simulink model "Battery_charge_discharge_FSBB_DCDC"  (R2022b)
settings: Solver=ode23tb  StartTime=0.0  StopTime=1.5  RelTol=1e-3  EnableMultiTasking=on
values from neighbouring files (symbols this model uses):
  time_step = 1 / wave_freq    (= 1.11111111111e-05)    [Battery_charge_discharge_FSBB_param_init.m]
undefined symbols (not defined in the file or in its folder): Ion, Lithium
libraries: spsTriangleGeneratorLib x13, spsSeriesRLCBranchLib x9, slpidlib x9, spsVoltageMeasurementLib x5, spsCurrentMeasurementLib x4, spsIGBTDiodeLib x4, spsBatteryLib x2, spsIdealSwitchLib x2, spsDCVoltageSourceLib x2, spsControlledVoltageSourceLib x1, spspowerguiLib x1
(part 2 of 2)

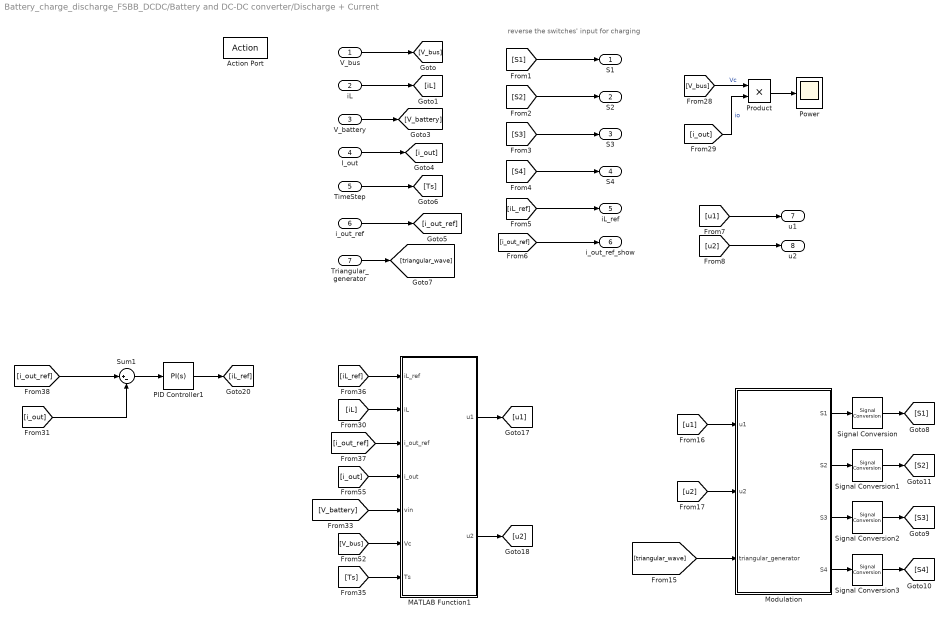
== system Battery_charge_discharge_FSBB_DCDC/Battery and DC-DC converter/Discharge + Current ==
  note: reverse the switches' input for charging
  V_bus : Inport
  iL : Inport  Port=2
  V_battery : Inport  Port=3
  I_out : Inport  Port=4
  TimeStep : Inport  Port=5
  i_out_ref : Inport  Port=6
  Triangular_generator : Inport  Port=7
  Action Port : ActionPort  ActionPortLabel=elseif( u1==1 & u2==1)
  MATLAB Function1 : MATLAB Function  TreatAsAtomicUnit=on
  Modulation : Subsystem
  PID Controller1 : slpidlib/PID Controller  Controller=PI  Form=Parallel  TimeDomain=Continuous-time  UseExternalTs=off  SampleTime=-1  IntegratorMethod=Forward Euler  FilterMethod=Forward Euler  ControllerParametersSource=internal  P=15  I=1000  UseKiTs=on  D=0  N=100  UseFilter=on  TunerSelectOption=Transfer Function Based (PID Tuner App)  InitialConditionSource=internal  InitialConditionForIntegrator=0  InitialConditionForFilter=0  DifferentiatorICPrevScaledInput=0  ExternalReset=none  TrackingMode=off  Kt=1  LimitOutput=on  SatLimitsSource=internal  UpperSaturationLimit=50  LowerSaturationLimit=-10  LinearizeAsGain=on  AntiWindupMode=none  Kb=1  LimitIntegrator=off  UpperIntegratorSaturationLimit=inf  LowerIntegratorSaturationLimit=-inf  POutMin=[]  POutMax=[]  IOutMin=[]  IOutMax=[]  DOutMin=[]  DOutMax=[]  NOutMin=[]  NOutMax=[]  SumOutMin=[]  SumOutMax=[]  SaturationOutMin=[]  SaturationOutMax=[]  PParamMin=[]  PParamMax=[]  IParamMin=[]  IParamMax=[]  DParamMin=[]  DParamMax=[]  NParamMin=[]  NParamMax=[]  KbParamMin=[]  KbParamMax=[]  KtParamMin=[]  KtParamMax=[]  KbOutMin=[]  KbOutMax=[]  KtOutMin=[]  KtOutMax=[]  IntegratorOutMin=[]  IntegratorOutMax=[]  FilterOutMin=[]  FilterOutMax=[]  SumI1OutMin=[]  SumI1OutMax=[]  SumI2OutMin=[]  SumI2OutMax=[]  SumI3OutMin=[]  SumI3OutMax=[]  SumI4OutMin=[]  SumI4OutMax=[]  SumDOutMin=[]  SumDOutMax=[]  DifferentiatorOutMin=[]  DifferentiatorOutMax=[]  FilterDiffOutCoefMin=[]  FilterDiffOutCoefMax=[]  ReciprocalOutMin=[]  ReciprocalOutMax=[]  SumDenOutMin=[]  SumDenOutMax=[]  SumNumOutMin=[]  SumNumOutMax=[]  DivideOutMin=[]  DivideOutMax=[]  UdiffTsProdOutMin=[]  UdiffTsProdOutMax=[]  NTsProdOutMin=[]  NTsProdOutMax=[]  UintegralTsProdOutMin=[]  UintegralTsProdOutMax=[]  UngainTsProdOutMin=[]  UngainTsProdOutMax=[]  ClampingZeroOutDataTypeStr=Inherit: Inherit via back propagation  ClampingZeroOutMin=[]  ClampingZeroOutMax=[]  FilterDenConstantOutDataTypeStr=Inherit: Inherit via back propagation  FilterDenConstantOutMin=[]  FilterDenConstantOutMax=[]  PCopyOutDataTypeStr=Inherit: Inherit via back propagation  PCopyOutMin=[]  PCopyOutMax=[]  NCopyOutDataTypeStr=Inherit: Inherit via back propagation  NCopyOutMin=[]  NCopyOutMax=[]  IntegratorContinuousStateAttributes=''  IntegratorStateMustResolveToSignalObject=off  IntegratorRTWStateStorageClass=Auto  FilterContinuousStateAttributes=''  FilterStateMustResolveToSignalObject=off  FilterRTWStateStorageClass=Auto  ParallelPVariant=InternalParameters  IdealPVariant=Disabled  IVariant=InternalParameters  DVariant=Disabled  IntegratorVariant=Continuous  SatVariant=Enabled  AWVariant=Passthrough  PCopyVariant=Disabled  TRVariant=Disabled  FdbkBlocksVariant=Forward  IdealPFdbkVariant=Disabled  SatFdbkVariant=Disabled  DerivativeFilterVariant=Disabled  NVariant=Disabled  NCopyVariant=Disabled_SignalSpec  FilterICVariant=Disabled  IntegratorICVariant=InternalICs  ExternalResetVariant=Disabled  TRSumVariant=Passthrough  SumFdbkVariant=Disabled  SumVariant=Sum_PI  TsampFilterVariant=InternalTs  TsampNgainVariant=Passthrough  TsampIntegralVariant=Passthrough  ExternalSaturationOutDataTypeStr=Inherit: Same as second input
  Power : Scope
  Product : Product
  Signal Conversion{,1..3} (4 alike) : SignalConversion  OverrideOpt=off
  Sum1 : Sum  Inputs=|+-
  S1 : Outport
  S2 : Outport  Port=2
  S3 : Outport  Port=3
  S4 : Outport  Port=4
  iL_ref : Outport  Port=5
  i_out_ref_show : Outport  Port=6
  u1 : Outport  Port=7
  u2 : Outport  Port=8
  wires:
  Modulation/2(S2) -> Signal Conversion1/1
  Modulation/1(S1) -> Signal Conversion/1
  Modulation/3(S3) -> Signal Conversion2/1
  [u1] -> Modulation/1(u1)
  [i_out] -> Product/2  "io"
  [u2] -> Modulation/2(u2)
  [V_bus] -> Product/1  "Vc"
  Product/1 -> Power/1
  Modulation/4(S4) -> Signal Conversion3/1
  V_bus/1 -> [V_bus]
  iL/1 -> [iL]
  V_battery/1 -> [V_battery]
  I_out/1 -> [i_out]
  TimeStep/1 -> [Ts]
  i_out_ref/1 -> [i_out_ref]
  [iL_ref] -> iL_ref/1
  [i_out_ref] -> i_out_ref_show/1
  [u2] -> u2/1
  [u1] -> u1/1
  [triangular_wave] -> Modulation/3(triangular_generator)
  Triangular_generator/1 -> [triangular_wave]
  Signal Conversion/1 -> [S1]
  Signal Conversion1/1 -> [S2]
  Signal Conversion2/1 -> [S3]
  Signal Conversion3/1 -> [S4]
  [iL] -> MATLAB Function1/2(iL)
  Sum1/1 -> PID Controller1/1
  [i_out] -> Sum1/2
  [i_out] -> MATLAB Function1/4(i_out)
  [V_bus] -> MATLAB Function1/6(Vc)
  [Ts] -> MATLAB Function1/7(Ts)
  PID Controller1/1 -> [iL_ref]
  MATLAB Function1/2(u2) -> [u2]
  MATLAB Function1/1(u1) -> [u1]
  [i_out_ref] -> Sum1/1
  [i_out_ref] -> MATLAB Function1/3(i_out_ref)
  [iL_ref] -> MATLAB Function1/1(iL_ref)
  [V_battery] -> MATLAB Function1/5(vin)
  [S1] -> S1/1
  [S3] -> S3/1
  [S4] -> S4/1
  [S2] -> S2/1

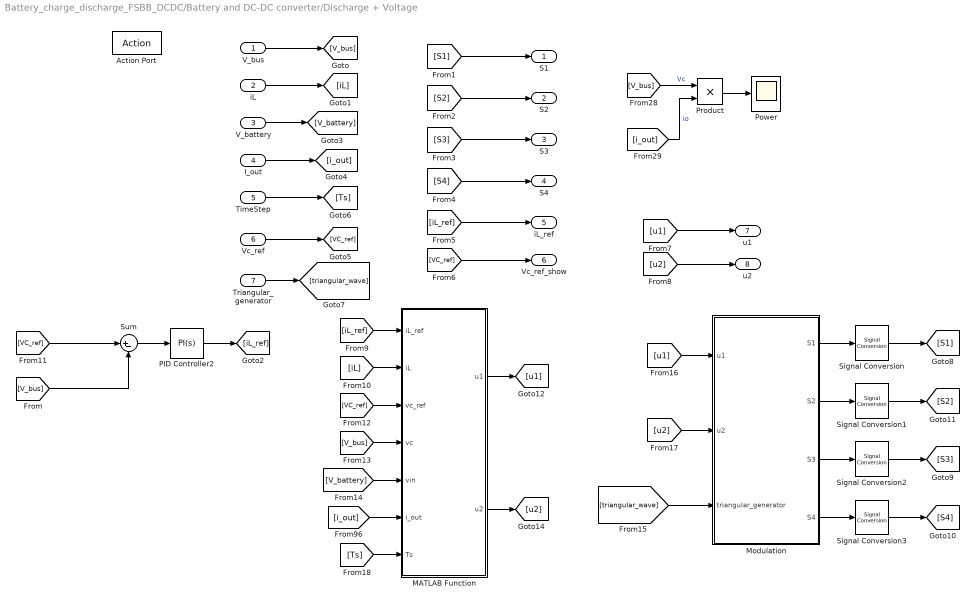
== system Battery_charge_discharge_FSBB_DCDC/Battery and DC-DC converter/Discharge + Voltage ==
  V_bus : Inport
  iL : Inport  Port=2
  V_battery : Inport  Port=3
  I_out : Inport  Port=4
  TimeStep : Inport  Port=5
  Vc_ref : Inport  Port=6
  Triangular_generator : Inport  Port=7
  Action Port : ActionPort  ActionPortLabel=if(u1 == 1 & u2 ==0)
  MATLAB Function : MATLAB Function  TreatAsAtomicUnit=on
  Modulation : Subsystem
  PID Controller2 : slpidlib/PID Controller  Controller=PI  Form=Parallel  TimeDomain=Continuous-time  UseExternalTs=off  SampleTime=-1  IntegratorMethod=Forward Euler  FilterMethod=Forward Euler  ControllerParametersSource=internal  P=15  I=1000  UseKiTs=on  D=0  N=100  UseFilter=on  TunerSelectOption=Transfer Function Based (PID Tuner App)  InitialConditionSource=internal  InitialConditionForIntegrator=0  InitialConditionForFilter=0  DifferentiatorICPrevScaledInput=0  ExternalReset=none  TrackingMode=off  Kt=1  LimitOutput=on  SatLimitsSource=internal  UpperSaturationLimit=50  LowerSaturationLimit=-10  LinearizeAsGain=on  AntiWindupMode=none  Kb=1  LimitIntegrator=off  UpperIntegratorSaturationLimit=inf  LowerIntegratorSaturationLimit=-inf  POutMin=[]  POutMax=[]  IOutMin=[]  IOutMax=[]  DOutMin=[]  DOutMax=[]  NOutMin=[]  NOutMax=[]  SumOutMin=[]  SumOutMax=[]  SaturationOutMin=[]  SaturationOutMax=[]  PParamMin=[]  PParamMax=[]  IParamMin=[]  IParamMax=[]  DParamMin=[]  DParamMax=[]  NParamMin=[]  NParamMax=[]  KbParamMin=[]  KbParamMax=[]  KtParamMin=[]  KtParamMax=[]  KbOutMin=[]  KbOutMax=[]  KtOutMin=[]  KtOutMax=[]  IntegratorOutMin=[]  IntegratorOutMax=[]  FilterOutMin=[]  FilterOutMax=[]  SumI1OutMin=[]  SumI1OutMax=[]  SumI2OutMin=[]  SumI2OutMax=[]  SumI3OutMin=[]  SumI3OutMax=[]  SumI4OutMin=[]  SumI4OutMax=[]  SumDOutMin=[]  SumDOutMax=[]  DifferentiatorOutMin=[]  DifferentiatorOutMax=[]  FilterDiffOutCoefMin=[]  FilterDiffOutCoefMax=[]  ReciprocalOutMin=[]  ReciprocalOutMax=[]  SumDenOutMin=[]  SumDenOutMax=[]  SumNumOutMin=[]  SumNumOutMax=[]  DivideOutMin=[]  DivideOutMax=[]  UdiffTsProdOutMin=[]  UdiffTsProdOutMax=[]  NTsProdOutMin=[]  NTsProdOutMax=[]  UintegralTsProdOutMin=[]  UintegralTsProdOutMax=[]  UngainTsProdOutMin=[]  UngainTsProdOutMax=[]  ClampingZeroOutDataTypeStr=Inherit: Inherit via back propagation  ClampingZeroOutMin=[]  ClampingZeroOutMax=[]  FilterDenConstantOutDataTypeStr=Inherit: Inherit via back propagation  FilterDenConstantOutMin=[]  FilterDenConstantOutMax=[]  PCopyOutDataTypeStr=Inherit: Inherit via back propagation  PCopyOutMin=[]  PCopyOutMax=[]  NCopyOutDataTypeStr=Inherit: Inherit via back propagation  NCopyOutMin=[]  NCopyOutMax=[]  IntegratorContinuousStateAttributes=''  IntegratorStateMustResolveToSignalObject=off  IntegratorRTWStateStorageClass=Auto  FilterContinuousStateAttributes=''  FilterStateMustResolveToSignalObject=off  FilterRTWStateStorageClass=Auto  ParallelPVariant=InternalParameters  IdealPVariant=Disabled  IVariant=InternalParameters  DVariant=Disabled  IntegratorVariant=Continuous  SatVariant=Enabled  AWVariant=Passthrough  PCopyVariant=Disabled  TRVariant=Disabled  FdbkBlocksVariant=Forward  IdealPFdbkVariant=Disabled  SatFdbkVariant=Disabled  DerivativeFilterVariant=Disabled  NVariant=Disabled  NCopyVariant=Disabled_SignalSpec  FilterICVariant=Disabled  IntegratorICVariant=InternalICs  ExternalResetVariant=Disabled  TRSumVariant=Passthrough  SumFdbkVariant=Disabled  SumVariant=Sum_PI  TsampFilterVariant=InternalTs  TsampNgainVariant=Passthrough  TsampIntegralVariant=Passthrough  ExternalSaturationOutDataTypeStr=Inherit: Same as second input
  Power : Scope
  Product : Product
  Signal Conversion{,1..3} (4 alike) : SignalConversion  OverrideOpt=off
  Sum : Sum  Inputs=|+-
  S1 : Outport
  S2 : Outport  Port=2
  S3 : Outport  Port=3
  S4 : Outport  Port=4
  iL_ref : Outport  Port=5
  Vc_ref_show : Outport  Port=6
  u1 : Outport  Port=7
  u2 : Outport  Port=8
  wires:
  PID Controller2/1 -> [iL_ref]
  Modulation/2(S2) -> Signal Conversion1/1
  [Ts] -> MATLAB Function/7(Ts)
  Modulation/1(S1) -> Signal Conversion/1
  Sum/1 -> PID Controller2/1
  Modulation/3(S3) -> Signal Conversion2/1
  MATLAB Function/2(u2) -> [u2]
  [V_bus] -> MATLAB Function/4(vc)
  [u1] -> Modulation/1(u1)
  [VC_ref] -> Sum/1
  [VC_ref] -> MATLAB Function/3(vc_ref)
  MATLAB Function/1(u1) -> [u1]
  [i_out] -> Product/2  "io"
  [u2] -> Modulation/2(u2)
  [i_out] -> MATLAB Function/6(i_out)
  [iL] -> MATLAB Function/2(iL)
  [V_battery] -> MATLAB Function/5(vin)
  [V_bus] -> Product/1  "Vc"
  [iL_ref] -> MATLAB Function/1(iL_ref)
  Product/1 -> Power/1
  Modulation/4(S4) -> Signal Conversion3/1
  V_bus/1 -> [V_bus]
  [V_bus] -> Sum/2
  iL/1 -> [iL]
  V_battery/1 -> [V_battery]
  I_out/1 -> [i_out]
  TimeStep/1 -> [Ts]
  [S1] -> S1/1
  [S2] -> S2/1
  [S4] -> S4/1
  [S3] -> S3/1
  Vc_ref/1 -> [VC_ref]
  [iL_ref] -> iL_ref/1
  [VC_ref] -> Vc_ref_show/1
  [u2] -> u2/1
  [u1] -> u1/1
  [triangular_wave] -> Modulation/3(triangular_generator)
  Triangular_generator/1 -> [triangular_wave]
  Signal Conversion/1 -> [S1]
  Signal Conversion1/1 -> [S2]
  Signal Conversion2/1 -> [S3]
  Signal Conversion3/1 -> [S4]

== system Battery_charge_discharge_FSBB_DCDC/Battery and DC-DC converter/If Action Subsystem ==
  Action Port : ActionPort  ActionPortLabel=else
  Constant : Constant
  Stop Simulation : Stop
  wires:
  Constant/1 -> Stop Simulation/1

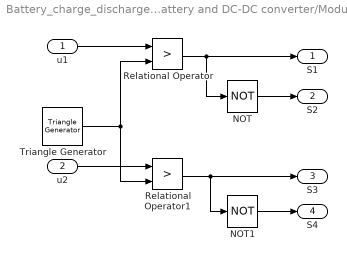
== system Battery_charge_discharge_FSBB_DCDC/Battery and DC-DC converter/Modulation ==
  u1 : Inport
  u2 : Inport  Port=2
  NOT : Logic  Operator=NOT  AllPortsSameDT=off  OutDataTypeStr=boolean
  NOT1 : Logic  Operator=NOT  AllPortsSameDT=off  OutDataTypeStr=boolean
  Relational Operator : RelationalOperator  Operator=>  OutDataTypeStr=boolean  RndMeth=Simplest  InputSameDT=off
  Relational Operator1 : RelationalOperator  Operator=>  OutDataTypeStr=boolean  RndMeth=Simplest  InputSameDT=off
  Triangle Generator : spsTriangleGeneratorLib/Triangle Generator  Freq=wave_freq  Phase=0  Ts=0
  S1 : Outport
  S2 : Outport  Port=2
  S3 : Outport  Port=3
  S4 : Outport  Port=4
  wires:
  u1/1 -> Relational Operator/1
  Triangle Generator/1 -> Relational Operator1/2, Relational Operator/2
  u2/1 -> Relational Operator1/1
  Relational Operator/1 -> NOT/1, S1/1
  NOT/1 -> S2/1
  Relational Operator1/1 -> NOT1/1, S3/1
  NOT1/1 -> S4/1

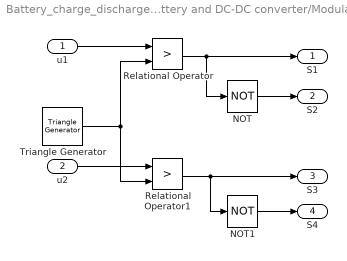
== system Battery_charge_discharge_FSBB_DCDC/Battery and DC-DC converter/Modulation1 ==
  u1 : Inport
  u2 : Inport  Port=2
  NOT : Logic  Operator=NOT  AllPortsSameDT=off  OutDataTypeStr=boolean
  NOT1 : Logic  Operator=NOT  AllPortsSameDT=off  OutDataTypeStr=boolean
  Relational Operator : RelationalOperator  Operator=>  OutDataTypeStr=boolean  RndMeth=Simplest  InputSameDT=off
  Relational Operator1 : RelationalOperator  Operator=>  OutDataTypeStr=boolean  RndMeth=Simplest  InputSameDT=off
  Triangle Generator : spsTriangleGeneratorLib/Triangle Generator  Freq=wave_freq  Phase=0  Ts=0
  S1 : Outport
  S2 : Outport  Port=2
  S3 : Outport  Port=3
  S4 : Outport  Port=4
  wires:
  u1/1 -> Relational Operator/1
  Triangle Generator/1 -> Relational Operator1/2, Relational Operator/2
  u2/1 -> Relational Operator1/1
  Relational Operator/1 -> NOT/1, S1/1
  NOT/1 -> S2/1
  Relational Operator1/1 -> NOT1/1, S3/1
  NOT1/1 -> S4/1

== system Battery_charge_discharge_FSBB_DCDC/Battery and DC-DC converter/Modulation2 ==
  u1 : Inport
  u2 : Inport  Port=2
  NOT : Logic  Operator=NOT  AllPortsSameDT=off  OutDataTypeStr=boolean
  NOT1 : Logic  Operator=NOT  AllPortsSameDT=off  OutDataTypeStr=boolean
  Relational Operator : RelationalOperator  Operator=>  OutDataTypeStr=boolean  RndMeth=Simplest  InputSameDT=off
  Relational Operator1 : RelationalOperator  Operator=>  OutDataTypeStr=boolean  RndMeth=Simplest  InputSameDT=off
  Triangle Generator : spsTriangleGeneratorLib/Triangle Generator  Freq=wave_freq  Phase=0  Ts=0
  S1 : Outport
  S2 : Outport  Port=2
  S3 : Outport  Port=3
  S4 : Outport  Port=4
  wires:
  u1/1 -> Relational Operator/1
  Triangle Generator/1 -> Relational Operator1/2, Relational Operator/2
  u2/1 -> Relational Operator1/1
  Relational Operator/1 -> NOT/1, S1/1
  NOT/1 -> S2/1
  Relational Operator1/1 -> NOT1/1, S3/1
  NOT1/1 -> S4/1

== system Battery_charge_discharge_FSBB_DCDC/Battery and DC-DC converter/Modulation3 ==
  u1 : Inport
  u2 : Inport  Port=2
  NOT : Logic  Operator=NOT  AllPortsSameDT=off  OutDataTypeStr=boolean
  NOT1 : Logic  Operator=NOT  AllPortsSameDT=off  OutDataTypeStr=boolean
  Relational Operator : RelationalOperator  Operator=>  OutDataTypeStr=boolean  RndMeth=Simplest  InputSameDT=off
  Relational Operator1 : RelationalOperator  Operator=>  OutDataTypeStr=boolean  RndMeth=Simplest  InputSameDT=off
  Triangle Generator : spsTriangleGeneratorLib/Triangle Generator  Freq=wave_freq  Phase=0  Ts=0
  S1 : Outport
  S2 : Outport  Port=2
  S3 : Outport  Port=3
  S4 : Outport  Port=4
  wires:
  u1/1 -> Relational Operator/1
  Triangle Generator/1 -> Relational Operator1/2, Relational Operator/2
  u2/1 -> Relational Operator1/1
  Relational Operator/1 -> NOT/1, S1/1
  NOT/1 -> S2/1
  Relational Operator1/1 -> NOT1/1, S3/1
  NOT1/1 -> S4/1

== system Battery_charge_discharge_FSBB_DCDC/Battery and DC-DC converter/Modulation5 ==
  u1 : Inport
  u2 : Inport  Port=2
  NOT : Logic  Operator=NOT  AllPortsSameDT=off  OutDataTypeStr=boolean
  NOT1 : Logic  Operator=NOT  AllPortsSameDT=off  OutDataTypeStr=boolean
  Relational Operator : RelationalOperator  Operator=>  OutDataTypeStr=boolean  RndMeth=Simplest  InputSameDT=off
  Relational Operator1 : RelationalOperator  Operator=>  OutDataTypeStr=boolean  RndMeth=Simplest  InputSameDT=off
  Triangle Generator : spsTriangleGeneratorLib/Triangle Generator  Freq=wave_freq  Phase=0  Ts=0
  S1 : Outport
  S2 : Outport  Port=2
  S3 : Outport  Port=3
  S4 : Outport  Port=4
  wires:
  u1/1 -> Relational Operator/1
  Triangle Generator/1 -> Relational Operator1/2, Relational Operator/2
  u2/1 -> Relational Operator1/1
  Relational Operator/1 -> NOT/1, S1/1
  NOT/1 -> S2/1
  Relational Operator1/1 -> NOT1/1, S3/1
  NOT1/1 -> S4/1

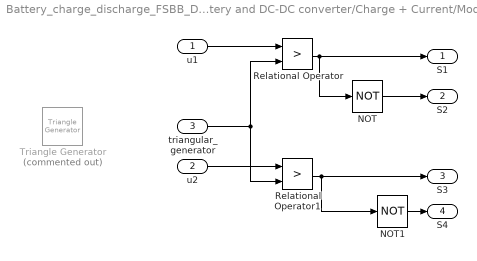
== system Battery_charge_discharge_FSBB_DCDC/Battery and DC-DC converter/Charge + Current/Modulation ==
  u1 : Inport
  u2 : Inport  Port=2
  triangular_generator : Inport  Port=3
  NOT : Logic  Operator=NOT  AllPortsSameDT=off  OutDataTypeStr=boolean
  NOT1 : Logic  Operator=NOT  AllPortsSameDT=off  OutDataTypeStr=boolean
  Relational Operator : RelationalOperator  Operator=>  OutDataTypeStr=boolean  RndMeth=Simplest  InputSameDT=off
  Relational Operator1 : RelationalOperator  Operator=>  OutDataTypeStr=boolean  RndMeth=Simplest  InputSameDT=off
  Triangle Generator : spsTriangleGeneratorLib/Triangle Generator  Commented=on  Freq=wave_freq  Phase=0  Ts=0
  S1 : Outport
  S2 : Outport  Port=2
  S3 : Outport  Port=3
  S4 : Outport  Port=4
  wires:
  u1/1 -> Relational Operator/1
  triangular_generator/1 -> Relational Operator1/2, Relational Operator/2
  u2/1 -> Relational Operator1/1
  NOT1/1 -> S4/1
  Relational Operator/1 -> S1/1, NOT/1
  Relational Operator1/1 -> S3/1, NOT1/1
  NOT/1 -> S2/1

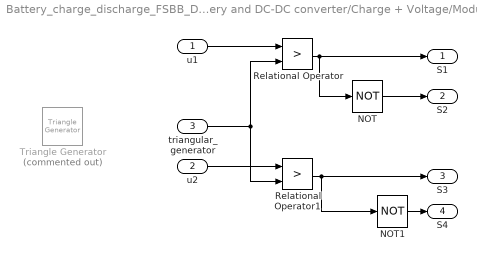
== system Battery_charge_discharge_FSBB_DCDC/Battery and DC-DC converter/Charge + Voltage/Modulation ==
  u1 : Inport
  u2 : Inport  Port=2
  triangular_generator : Inport  Port=3
  NOT : Logic  Operator=NOT  AllPortsSameDT=off  OutDataTypeStr=boolean
  NOT1 : Logic  Operator=NOT  AllPortsSameDT=off  OutDataTypeStr=boolean
  Relational Operator : RelationalOperator  Operator=>  OutDataTypeStr=boolean  RndMeth=Simplest  InputSameDT=off
  Relational Operator1 : RelationalOperator  Operator=>  OutDataTypeStr=boolean  RndMeth=Simplest  InputSameDT=off
  Triangle Generator : spsTriangleGeneratorLib/Triangle Generator  Commented=on  Freq=wave_freq  Phase=0  Ts=0
  S1 : Outport
  S2 : Outport  Port=2
  S3 : Outport  Port=3
  S4 : Outport  Port=4
  wires:
  u1/1 -> Relational Operator/1
  triangular_generator/1 -> Relational Operator1/2, Relational Operator/2
  u2/1 -> Relational Operator1/1
  NOT1/1 -> S4/1
  Relational Operator/1 -> S1/1, NOT/1
  Relational Operator1/1 -> S3/1, NOT1/1
  NOT/1 -> S2/1

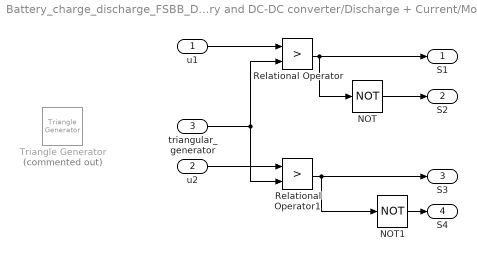
== system Battery_charge_discharge_FSBB_DCDC/Battery and DC-DC converter/Discharge + Current/Modulation ==
  u1 : Inport
  u2 : Inport  Port=2
  triangular_generator : Inport  Port=3
  NOT : Logic  Operator=NOT  AllPortsSameDT=off  OutDataTypeStr=boolean
  NOT1 : Logic  Operator=NOT  AllPortsSameDT=off  OutDataTypeStr=boolean
  Relational Operator : RelationalOperator  Operator=>  OutDataTypeStr=boolean  RndMeth=Simplest  InputSameDT=off
  Relational Operator1 : RelationalOperator  Operator=>  OutDataTypeStr=boolean  RndMeth=Simplest  InputSameDT=off
  Triangle Generator : spsTriangleGeneratorLib/Triangle Generator  Commented=on  Freq=wave_freq  Phase=0  Ts=0
  S1 : Outport
  S2 : Outport  Port=2
  S3 : Outport  Port=3
  S4 : Outport  Port=4
  wires:
  u1/1 -> Relational Operator/1
  triangular_generator/1 -> Relational Operator1/2, Relational Operator/2
  u2/1 -> Relational Operator1/1
  NOT1/1 -> S4/1
  Relational Operator/1 -> S1/1, NOT/1
  Relational Operator1/1 -> S3/1, NOT1/1
  NOT/1 -> S2/1

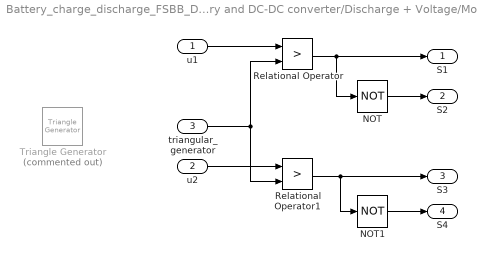
== system Battery_charge_discharge_FSBB_DCDC/Battery and DC-DC converter/Discharge + Voltage/Modulation ==
  u1 : Inport
  u2 : Inport  Port=2
  triangular_generator : Inport  Port=3
  NOT : Logic  Operator=NOT  AllPortsSameDT=off  OutDataTypeStr=boolean
  NOT1 : Logic  Operator=NOT  AllPortsSameDT=off  OutDataTypeStr=boolean
  Relational Operator : RelationalOperator  Operator=>  OutDataTypeStr=boolean  RndMeth=Simplest  InputSameDT=off
  Relational Operator1 : RelationalOperator  Operator=>  OutDataTypeStr=boolean  RndMeth=Simplest  InputSameDT=off
  Triangle Generator : spsTriangleGeneratorLib/Triangle Generator  Commented=on  Freq=wave_freq  Phase=0  Ts=0
  S1 : Outport
  S2 : Outport  Port=2
  S3 : Outport  Port=3
  S4 : Outport  Port=4
  wires:
  u1/1 -> Relational Operator/1
  triangular_generator/1 -> Relational Operator1/2, Relational Operator/2
  u2/1 -> Relational Operator1/1
  Relational Operator/1 -> NOT/1, S1/1
  NOT/1 -> S2/1
  Relational Operator1/1 -> NOT1/1, S3/1
  NOT1/1 -> S4/1

== matlab function Battery_charge_discharge_FSBB_DCDC/Battery and DC-DC converter/Discharge + Current/MATLAB Function1 ==
  settings: updateMethod=DISCRETE
  data: iL_ref input; u1 output; iL input; i_out_ref input; i_out input; vin input; Vc input; Ts input; u2 output
function [u1, u2] = Passivity_BC(iL_ref, iL,i_out_ref, i_out, vin, Vc, Ts)
% Constant output current Module
% param iL: inductor's current
% param iL_ref: expected value of inductor's current
% param i_out: dcdc output current 
% param i_out_ref
% param vin: input voltage
% param Vc: output voltage
%% system parameters
L = 2000e-6;  % Inductance 电感 20uH
RL = 0.004;
C_output = 1440e-6;  % 电容大小

zeta1 = 6;  % dumping gains
zeta2 = 0.08;

% error functions: state variable
x1 = iL - iL_ref;
x2 = i_out - i_out_ref;
persistent iL_ref_old Vc_old;
if isempty(iL_ref_old)
    iL_ref_old = 0;
    Vc_old = 0;
end

diL_ref = (iL_ref - iL_ref_old) / Ts;
dVc_ref = (Vc - Vc_old) / Ts;
%% calculate switching signal: u1,u2
u2 = 1 / iL_ref * (iL_ref - C_output * dVc_ref - i_out_ref + x2*zeta2);
u1 = 1 / vin * (L*diL_ref + RL * iL_ref + Vc * (1 - u2) - x1*zeta1);

iL_ref_old = iL_ref;
Vc_old = Vc;

== matlab function Battery_charge_discharge_FSBB_DCDC/Battery and DC-DC converter/Charge + Current/MATLAB Function2 ==
  settings: updateMethod=DISCRETE
  data: iL_ref input; u1 output; iL input; i_out_ref input; i_out input; vin input; Vc input; Ts input; u2 output
function [u1, u2] = Passivity_BC(iL_ref, iL,i_out_ref, i_out, vin, Vc, Ts)
% Constant output current Module
% param iL: inductor's current
% param iL_ref: expected value of inductor's current
% param i_out: dcdc output current 
% param i_out_ref
% param vin: input voltage
% param Vc: output voltage
%% system parameters
L = 20e-6;  % Inductance 电感 20uH
RL = 0.004;
C_output = 1440e-6;  % 电容大小

zeta1 = 6;  % dumping gains
zeta2 = 0.08;

% error functions: state variable
x1 = iL - iL_ref;
x2 = i_out - i_out_ref;
persistent iL_ref_old Vc_old;
if isempty(iL_ref_old)
    iL_ref_old = 0;
    Vc_old = 0;
end

diL_ref = (iL_ref - iL_ref_old) / Ts;
dVc_ref = (Vc - Vc_old) / Ts;
%% calculate switching signal: u1,u2
u2 = 1 / iL_ref * (iL_ref - C_output * dVc_ref - i_out_ref + x2*zeta2);
u1 = 1 / vin * (L*diL_ref + RL * iL_ref + Vc * (1 - u2) - x1*zeta1);

iL_ref_old = iL_ref;
Vc_old = Vc;

== matlab function Battery_charge_discharge_FSBB_DCDC/Battery and DC-DC converter/MATLAB Function1 ==
  settings: updateMethod=DISCRETE
  data: iL_ref input; u1 output; iL input; i_out_ref input; i_out input; vin input; Vc input; Ts input; u2 output
function [u1, u2] = Passivity_BC(iL_ref, iL,i_out_ref, i_out, vin, Vc, Ts)
% Constant output current Module
% param iL: inductor's current
% param iL_ref: expected value of inductor's current
% param i_out: dcdc output current 
% param i_out_ref
% param vin: input voltage
% param Vc: output voltage
%% system parameters
L = 2000e-6;  % Inductance 电感 20uH
RL = 0.004;
C_output = 1440e-6;  % 电容大小

zeta1 = 6;  % dumping gains
zeta2 = 0.08;

% error functions: state variable
x1 = iL - iL_ref;
x2 = i_out - i_out_ref;
persistent iL_ref_old Vc_old;
if isempty(iL_ref_old)
    iL_ref_old = 0;
    Vc_old = 0;
end

diL_ref = (iL_ref - iL_ref_old) / Ts;
dVc_ref = (Vc - Vc_old) / Ts;
%% calculate switching signal: u1,u2
u2 = 1 / iL_ref * (iL_ref - C_output * dVc_ref - i_out_ref + x2*zeta2);
u1 = 1 / vin * (L*diL_ref + RL * iL_ref + Vc * (1 - u2) - x1*zeta1);

iL_ref_old = iL_ref;
Vc_old = Vc;

== matlab function Battery_charge_discharge_FSBB_DCDC/Battery and DC-DC converter/MATLAB Function ==
  settings: updateMethod=DISCRETE
  data: iL_ref input; u1 output; iL input; vc_ref input; vc input; vin input; i_out input; Ts input; u2 output
function [u1, u2] = Passivity_BC(iL_ref, iL, vc_ref, vc, vin, i_out, Ts)
% Constant output voltage Module
%   param vc_ref: expected
%   param vc: dcdc output voltage
%   param vin: input voltage
%   param io: current in output side
%% system parameters
L = 20e-6;  % Inductance 电感 20uH
RL = 0.004;
Co = 1440e-6;  % 电容大小

zeta1 = 6;  % dumping gains
zeta2 = 0.08; 

% error functions: state variable
x1 = iL - iL_ref;
x2 = vc - vc_ref;
persistent iL_ref_old vc_ref_old;
if isempty(iL_ref_old)
    iL_ref_old = 0;
    vc_ref_old = 0;
end

diL_ref = (iL_ref - iL_ref_old) / Ts;
dvc_ref = (vc_ref - vc_ref_old) / Ts;
%% calculate switching signal: u1,u2
u2 = 1 / iL_ref * (iL_ref - dvc_ref * Co - i_out + x2*zeta2);
u1 = 1 / vin * (L*diL_ref + RL*iL_ref + vc_ref*(1-u2) - x1*zeta1);
iL_ref_old = iL_ref;
vc_ref_old = vc_ref;

== matlab function Battery_charge_discharge_FSBB_DCDC/Battery and DC-DC converter/MATLAB Function2 ==
  settings: updateMethod=DISCRETE
  data: iL_ref input; u1 output; iL input; i_out_ref input; i_out input; vin input; Vc input; Ts input; u2 output
function [u1, u2] = Passivity_BC(iL_ref, iL,i_out_ref, i_out, vin, Vc, Ts)
% Constant output current Module
% param iL: inductor's current
% param iL_ref: expected value of inductor's current
% param i_out: dcdc output current 
% param i_out_ref
% param vin: input voltage
% param Vc: output voltage
%% system parameters
L = 20e-6;  % Inductance 电感 20uH
RL = 0.004;
C_output = 1440e-6;  % 电容大小

zeta1 = 6;  % dumping gains
zeta2 = 0.08;

% error functions: state variable
x1 = iL - iL_ref;
x2 = i_out - i_out_ref;
persistent iL_ref_old Vc_old;
if isempty(iL_ref_old)
    iL_ref_old = 0;
    Vc_old = 0;
end

diL_ref = (iL_ref - iL_ref_old) / Ts;
dVc_ref = (Vc - Vc_old) / Ts;
%% calculate switching signal: u1,u2
u2 = 1 / iL_ref * (iL_ref - C_output * dVc_ref - i_out_ref + x2*zeta2);
u1 = 1 / vin * (L*diL_ref + RL * iL_ref + Vc * (1 - u2) - x1*zeta1);

iL_ref_old = iL_ref;
Vc_old = Vc;

== matlab function Battery_charge_discharge_FSBB_DCDC/Battery and DC-DC converter/MATLAB Function3 ==
  settings: updateMethod=DISCRETE
  data: iL_ref input; u1 output; iL input; vc_ref input; vc input; vin input; i_out input; Ts input; u2 output
function [u1, u2] = Passivity_BC(iL_ref, iL, vc_ref, vc, vin, i_out, Ts)
% Constant output voltage Module
%   param vc_ref: expected
%   param vc: dcdc output voltage
%   param vin: input voltage
%   param io: current in output side
%% system parameters
L = 20e-6;  % Inductance 电感 20uH
RL = 0.004;
Co = 1440e-6;  % 电容大小

zeta1 = 6;  % dumping gains
zeta2 = 0.08; 

% error functions: state variable
x1 = iL - iL_ref;
x2 = vc - vc_ref;
persistent iL_ref_old vc_ref_old;
if isempty(iL_ref_old)
    iL_ref_old = 0;
    vc_ref_old = 0;
end

diL_ref = (iL_ref - iL_ref_old) / Ts;
dvc_ref = (vc_ref - vc_ref_old) / Ts;
%% calculate switching signal: u1,u2
u2 = 1 / iL_ref * (iL_ref - dvc_ref * Co - i_out + x2*zeta2);
u1 = 1 / vin * (L*diL_ref + RL*iL_ref + vc_ref*(1-u2) - x1*zeta1);
iL_ref_old = iL_ref;
vc_ref_old = vc_ref;

== matlab function Battery_charge_discharge_FSBB_DCDC/Battery and DC-DC converter/Discharge + Voltage/MATLAB Function ==
  settings: updateMethod=DISCRETE
  data: iL_ref input; u1 output; iL input; vc_ref input; vc input; vin input; i_out input; Ts input; u2 output
function [u1, u2] = Passivity_BC(iL_ref, iL, vc_ref, vc, vin, i_out, Ts)
% Constant output voltage Module
%   param vc_ref: expected
%   param vc: dcdc output voltage
%   param vin: input voltage
%   param io: current in output side
%% system parameters
L = 20e-6;  % Inductance 电感 20uH
RL = 0.004;
Co = 1440e-6;  % 电容大小

zeta1 = 6;  % dumping gains
zeta2 = 0.08; 

% error functions: state variable
x1 = iL - iL_ref;
x2 = vc - vc_ref;
persistent iL_ref_old vc_ref_old;
if isempty(iL_ref_old)
    iL_ref_old = 0;
    vc_ref_old = 0;
end

diL_ref = (iL_ref - iL_ref_old) / Ts;
dvc_ref = (vc_ref - vc_ref_old) / Ts;
%% calculate switching signal: u1,u2
u2 = 1 / iL_ref * (iL_ref - dvc_ref * Co - i_out + x2*zeta2);
u1 = 1 / vin * (L*diL_ref + RL*iL_ref + vc_ref*(1-u2) - x1*zeta1);
iL_ref_old = iL_ref;
vc_ref_old = vc_ref;

== matlab function Battery_charge_discharge_FSBB_DCDC/Battery and DC-DC converter/MATLAB Function5 ==
  settings: updateMethod=DISCRETE
  data: iL_ref input; u1 output; iL input; i_out_ref input; i_out input; vin input; Vc input; Ts input; u2 output
function [u1, u2] = Passivity_BC(iL_ref, iL,i_out_ref, i_out, vin, Vc, Ts)
% Constant output current Module
% param iL: inductor's current
% param iL_ref: expected value of inductor's current
% param i_out: dcdc output current 
% param i_out_ref
% param vin: input voltage
% param Vc: output voltage
%% system parameters
L = 2000e-6;  % Inductance 电感 20uH
RL = 0.004;
C_output = 1440e-6;  % 电容大小

zeta1 = 6;  % dumping gains
zeta2 = 0.08;

% error functions: state variable
x1 = iL - iL_ref;
x2 = i_out - i_out_ref;
persistent iL_ref_old Vc_old;
if isempty(iL_ref_old)
    iL_ref_old = 0;
    Vc_old = 0;
end

diL_ref = (iL_ref - iL_ref_old) / Ts;
dVc_ref = (Vc - Vc_old) / Ts;
%% calculate switching signal: u1,u2
u2 = 1 / iL_ref * (iL_ref - C_output * dVc_ref - i_out_ref + x2*zeta2);
u1 = 1 / vin * (L*diL_ref + RL * iL_ref + Vc * (1 - u2) - x1*zeta1);

iL_ref_old = iL_ref;
Vc_old = Vc;

== matlab function Battery_charge_discharge_FSBB_DCDC/Battery and DC-DC converter/Charge + Voltage/MATLAB Function3 ==
  settings: updateMethod=DISCRETE
  data: iL_ref input; u1 output; iL input; vc_ref input; vc input; vin input; i_out input; Ts input; u2 output
function [u1, u2] = Passivity_BC(iL_ref, iL, vc_ref, vc, vin, i_out, Ts)
% Constant output voltage Module
%   param vc_ref: expected
%   param vc: dcdc output voltage
%   param vin: input voltage
%   param io: current in output side
%% system parameters
L = 20e-6;  % Inductance 电感 20uH
RL = 0.004;
Co = 1440e-6;  % 电容大小

zeta1 = 6;  % dumping gains
zeta2 = 0.08; 

% error functions: state variable
x1 = iL - iL_ref;
x2 = vc - vc_ref;
persistent iL_ref_old vc_ref_old;
if isempty(iL_ref_old)
    iL_ref_old = 0;
    vc_ref_old = 0;
end

diL_ref = (iL_ref - iL_ref_old) / Ts;
dvc_ref = (vc_ref - vc_ref_old) / Ts;
%% calculate switching signal: u1,u2
u2 = 1 / iL_ref * (iL_ref - dvc_ref * Co - i_out + x2*zeta2);
u1 = 1 / vin * (L*diL_ref + RL*iL_ref + vc_ref*(1-u2) - x1*zeta1);
iL_ref_old = iL_ref;
vc_ref_old = vc_ref;
